simulink model "MPC_control"  (R2018a)
settings: Solver=FixedStepAuto  StartTime=0  StopTime=Tend  FixedStep=0.001  RelTol=5e-3
model workspace (MAT data in the model file):
  A_mu = 10
  B_reff = 8.386
  Cz = 7766.25
  DCT_Param : struct (value not decoded)
  D_reff = 0.25826
  Downshift_Speeds = [9.5625 12.9375 16.3125 19.6875 23.0625 26.4375 29.8125 33.1875 36.5625 39.9375 43.3125 46.6875 ... (28 elements, 4x7)]
  Pedal_Positions = [0.1 0.4 0.5 0.9]
  SUS : struct (value not decoded)
  Upshift_Speeds = [12.9375 16.3125 19.6875 33 26.4375 29.8125 33.1875 52.5 39.9375 43.3125 46.6875 77.25 ... (28 elements, 4x7)]
  VEH : struct (value not decoded)
  V_o = 16.7
  V_xlow = 1
  WH : struct (value not decoded)
  a = 1.4
  alpha_max = 1.5
  alpha_min = -1.5
  b = 1.8
  c_zo = 209651
  epsilon = 0.1
  h = 0.134
  path : struct (value not decoded)
  pio = 220000
  q_Fcx = 0
  q_Fz2 = 15.4
  q_Fzy = 0
  q_reo = 0.9974
  q_sx1 = -0.007764
  q_sx10 = 0.2824
  q_sx11 = 5.349
  q_sx12 = 0
  q_sx13 = 0
  q_sx14 = 0
  q_sx2 = 1.1915
  q_sx3 = 0.013948
  q_sx4 = 4.912
  q_sx5 = 1.02
  q_sx6 = 22.83
  q_sx7 = 0.7104
  q_sx8 = -0.023393
  q_sx9 = 0.6581
  q_sy1 = 0.00702
  q_sy2 = 0
  q_sy3 = 0.001515
  q_sy4 = 8.514e-05
  q_sy5 = 0
  q_sy6 = 0
  q_sy7 = 0.9008
  q_sy8 = -0.4089
  q_v1 = 0.0007742
  q_v2 = 0.04667
  r_Bx1 = 12.531
  r_Bx2 = 9.532
  r_Bx3 = 0
  r_By1 = 10.615
  r_By2 = 7.705
  r_By3 = 3.433e-06
  r_By4 = 0
  r_Cx1 = 1.019
  r_Cy1 = 1.0585
  r_Ex1 = -0.4487
  r_Ex2 = -0.4726
  r_Ey1 = 0.3132
  r_Ey2 = 7.63e-06
  r_Hx1 = 0.0002374
  r_Hy1 = 0.011646
  r_Hy2 = 7.63e-06
  r_Vy1 = 0.05654
  r_Vy2 = 7.63e-06
  r_Vy3 = 0
  r_Vy4 = 99.9
  r_Vy5 = 2
  r_Vy6 = 15.814
  r_o = 0.3135
  vehWidth = 2
  w = 1
symbols that are objects in the model workspace (value not decoded): VEH
undefined symbols (not defined in the file): Cok_1, Cok_2, Cok_3, Cok_4, Cok_5, Cok_6, Cok_7, Cok_8, Cok_9, Cout_1, Cout_2, Cout_3, Cout_4, Cout_5, Cout_6, Cout_7, Cout_8, Cout_9, DiscIntNeverNeededParam, Dout_1, Dout_2, Dout_3, Dout_4, Dout_5, Dout_6, Dout_7, Dout_8, Dout_9, F_1, F_2, F_3, F_4, F_5, F_6, F_7, F_8, F_9, Gd_1, Gd_2, Gd_3, Gd_4, Gd_5, Gd_6, Gd_7, Gd_8, Gd_9, Gok_1, Gok_2, Gok_3, Gok_4, Gok_5, Gok_6, Gok_7, Gok_8, Gok_9, Gsys_2, Gsys_9, Hd_1, Hd_2, Hd_3 ... (+70)
libraries: robotalgslib x10, simulink x5, sim3dlib x2, autolibutils x1, vehdynlibviscommon x1
(part 3 of 5)

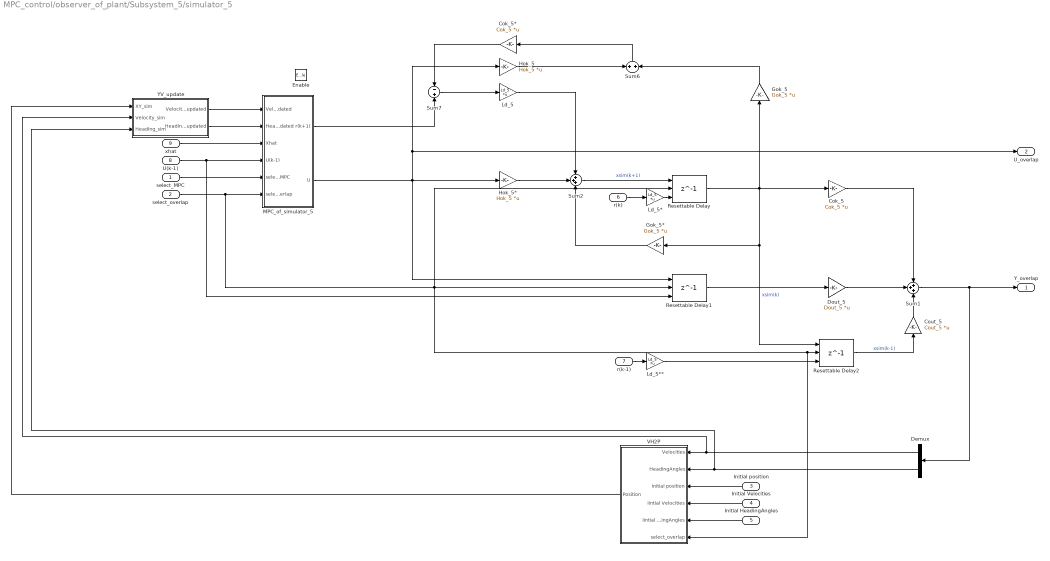
== system MPC_control/observer_of_plant/Subsystem_5/simulator_5 ==
  select_MPC : Inport
  select_overlap : Inport  Port=2
  Initial position : Inport  Port=3
  Initial Velocities : Inport  Port=4
  Initial HeadingAngles : Inport  Port=5
  r(k) : Inport  Port=6
  r(k-1) : Inport  Port=7
  U(k-1) : Inport  Port=8
  xhat : Inport  Port=9
  Enable : EnablePort
  Cok_5 : Gain  Gain=Cok_5  Multiplication=Matrix(K*u) (u vector)
  Cok_5* : Gain  Gain=Cok_5  Multiplication=Matrix(K*u) (u vector)
  Cout_5 : Gain  Gain=Cout_5  Multiplication=Matrix(K*u) (u vector)
  Demux : Demux  Outputs=2
  Dout_5 : Gain  Gain=Dout_5  Multiplication=Matrix(K*u) (u vector)
  Gok_5 : Gain  Gain=Gok_5  Multiplication=Matrix(K*u) (u vector)
  Gok_5* : Gain  Gain=Gok_5  Multiplication=Matrix(K*u) (u vector)
  Hok_5 : Gain  Gain=Hok_5  Multiplication=Matrix(K*u) (u vector)
  Hok_5* : Gain  Gain=Hok_5  Multiplication=Matrix(K*u) (u vector)
  Ld_5 : Gain  Gain=Ld_5  Multiplication=Matrix(K*u) (u vector)
  Ld_5* : Gain  Gain=Ld_5  Multiplication=Matrix(K*u) (u vector)
  Ld_5** : Gain  Gain=Ld_5  Multiplication=Matrix(K*u) (u vector)
  MPC_of_simulator_5 : Subsystem
  Resettable Delay : Delay  DelayLength=1  InitialConditionSource=Input port  ExternalReset=Rising  SampleTime=Ts
      settings: InputPortMap=u0,r5,p4
  Resettable Delay1 : Delay  DelayLength=1  InitialConditionSource=Input port  ExternalReset=Rising  SampleTime=Ts
      settings: InputPortMap=u0,r5,p4
  Resettable Delay2 : Delay  DelayLength=1  InitialConditionSource=Input port  ExternalReset=Rising  SampleTime=Ts
      settings: InputPortMap=u0,r5,p4
  Sum1 : Sum  Inputs=+++
  Sum2 : Sum  Inputs=+++
  Sum6 : Sum
  Sum7 : Sum  Inputs=-+
  VH2P : Subsystem
  YV_update : Subsystem  TreatAsAtomicUnit=on
  Y_overlap : Outport
  U_overlap : Outport  Port=2
  wires:
  Initial position/1 -> VH2P/3(Initial position)
  Sum2/1 -> Resettable Delay/1  "xsim(k+1)"
  Demux/2 -> VH2P/2(HeadingAngles), YV_update/3(Heading_sim)
  Ld_5/1 -> Sum2/1
  Sum7/1 -> Ld_5/1
  Cout_5/1 -> Sum1/3
  MPC_of_simulator_5/2(U) -> Hok_5*/1, Resettable Delay1/1, Hok_5/1, U_overlap/1
  Hok_5*/1 -> Sum2/2
  Gok_5*/1 -> Sum2/3
  Resettable Delay2/1 -> Cout_5/1  "xsim(k-1)"
  VH2P/1(Position) -> YV_update/1(XY_sim)
  Demux/1 -> YV_update/2(Velocity_sim), VH2P/1(Velocities)
  Resettable Delay/1 -> Gok_5*/1, Resettable Delay2/1, Gok_5/1, Cok_5/1  "xsim(k)"
  Hok_5/1 -> Sum6/1
  Sum6/1 -> Cok_5*/1
  Dout_5/1 -> Sum1/2
  Resettable Delay1/1 -> Dout_5/1
  Cok_5/1 -> Sum1/1
  YV_update/2(Heading_updated) -> MPC_of_simulator_5/2(Heading_updated)
  YV_update/1(Velocity_updated) -> MPC_of_simulator_5/1(Velocity_updated)
  r(k)/1 -> Ld_5*/1
  Ld_5*/1 -> Resettable Delay/3
  U(k-1)/1 -> MPC_of_simulator_5/4(U(k-1)), Resettable Delay1/3
  r(k-1)/1 -> Ld_5**/1
  Ld_5**/1 -> Resettable Delay2/3
  Initial Velocities/1 -> VH2P/4(Iintial Velocities)
  Initial HeadingAngles/1 -> VH2P/5(Iintial HeadingAngles)
  select_overlap/1 -> MPC_of_simulator_5/6(select_overlap), Resettable Delay/2, VH2P/6(select_overlap), Resettable Delay2/2, Resettable Delay1/2
  Gok_5/1 -> Sum6/2
  Cok_5*/1 -> Sum7/1
  select_MPC/1 -> MPC_of_simulator_5/5(select_MPC)
  Sum1/1 -> Y_overlap/1, Demux/1
  MPC_of_simulator_5/1(r(k+1)) -> Sum7/2
  xhat/1 -> MPC_of_simulator_5/3(Xhat)

== system MPC_control/observer_of_plant/Subsystem_6/observer_of_simulator_6 ==
  select_overlap : Inport
  U_overlap : Inport  Port=2
  U : Inport  Port=3
  U(k-1) : Inport  Port=4
  Y_overlap : Inport  Port=5
  Y : Inport  Port=6
  r(k-1) : Inport  Port=7
  Cok_6 : Gain  Gain=Cok_6  Multiplication=Matrix(K*u) (u vector)
  Cok_6* : Gain  Gain=Cok_6  Multiplication=Matrix(K*u) (u vector)
  Delay : Delay  DelayLength=1  InitialConditionSource=Input port  InitialCondition=0  ExternalReset=Rising  SampleTime=Ts
      settings: InputPortMap=u0,r5,p4
  Delay1 : Delay  DelayLength=1  InitialConditionSource=Input port  InitialCondition=0  ExternalReset=Rising  SampleTime=Ts
      settings: InputPortMap=u0,r5,p4
  Gd_6 : Gain  Gain=Gd_6  Multiplication=Matrix(K*u) (u vector)
  Gok_6 : Gain  Gain=Gok_6  Multiplication=Matrix(K*u) (u vector)
  Hd_6 : Gain  Gain=Hd_6  Multiplication=Matrix(K*u) (u vector)
  Hok_6 : Gain  Gain=Hok_6  Multiplication=Matrix(K*u) (u vector)
  Ld_6 : Gain  Gain=Ld_6  Multiplication=Matrix(K*u) (u vector)
  Ld_6* : Gain  Gain=Ld_6  Multiplication=Matrix(K*u) (u vector)
  Sum : Sum  Inputs=|-+
  Sum1 : Sum
  Sum2 : Sum  Inputs=|-+
  Sum4 : Sum  Inputs=+++
  Switch1 : Switch  Threshold=1
  Switch2 : Switch  Threshold=1
  xhat : Outport
  sye : Outport  Port=2
  ope : Outport  Port=3
  wires:
  Hd_6/1 -> Sum4/2
  Ld_6/1 -> Sum4/1
  Delay1/1 -> Hok_6/1, Hd_6/1
  U_overlap/1 -> Switch2/1
  Gd_6/1 -> Sum4/3
  U/1 -> Switch2/3
  Delay/1 -> Gok_6/1, Gd_6/1
  Y_overlap/1 -> Switch1/1
  U(k-1)/1 -> Delay1/3
  select_overlap/1 -> Delay/2, Delay1/2, Switch2/2, Switch1/2
  r(k-1)/1 -> Ld_6*/1
  Switch1/1 -> Ld_6/1
  Switch2/1 -> Delay1/1
  Ld_6*/1 -> Delay/3
  Sum2/1 -> sye/1
  Gok_6/1 -> Sum1/1
  Cok_6/1 -> Sum/1
  Hok_6/1 -> Sum1/2
  Y/1 -> Sum/2, Sum2/2, Switch1/3
  Cok_6*/1 -> Sum2/1
  Sum1/1 -> Cok_6*/1
  Sum/1 -> ope/1
  Sum4/1 -> xhat/1, Cok_6/1, Delay/1  "xhat"

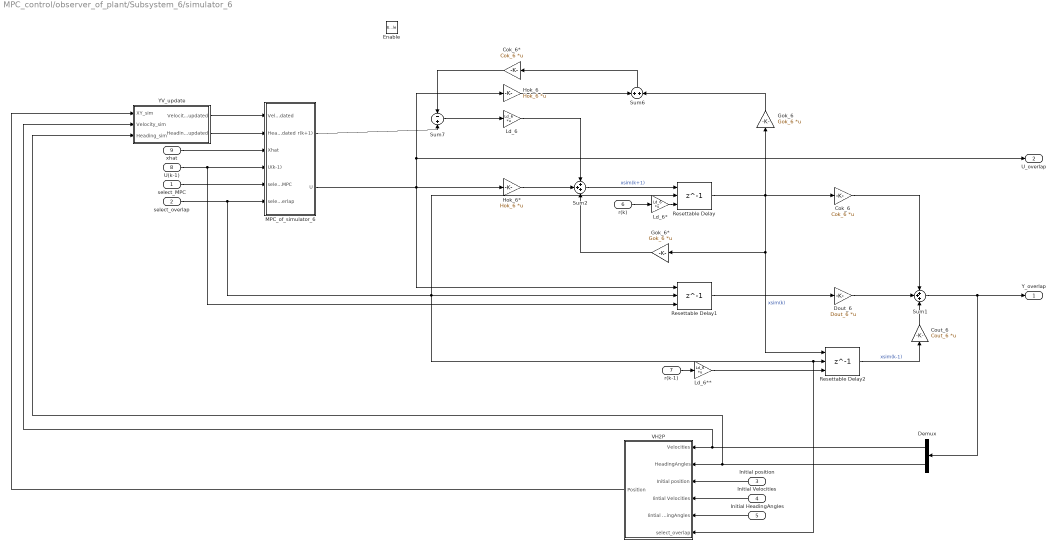
== system MPC_control/observer_of_plant/Subsystem_6/simulator_6 ==
  select_MPC : Inport
  select_overlap : Inport  Port=2
  Initial position : Inport  Port=3
  Initial Velocities : Inport  Port=4
  Initial HeadingAngles : Inport  Port=5
  r(k) : Inport  Port=6
  r(k-1) : Inport  Port=7
  U(k-1) : Inport  Port=8
  xhat : Inport  Port=9
  Enable : EnablePort
  Cok_6 : Gain  Gain=Cok_6  Multiplication=Matrix(K*u) (u vector)
  Cok_6* : Gain  Gain=Cok_6  Multiplication=Matrix(K*u) (u vector)
  Cout_6 : Gain  Gain=Cout_6  Multiplication=Matrix(K*u) (u vector)
  Demux : Demux  Outputs=2
  Dout_6 : Gain  Gain=Dout_6  Multiplication=Matrix(K*u) (u vector)
  Gok_6 : Gain  Gain=Gok_6  Multiplication=Matrix(K*u) (u vector)
  Gok_6* : Gain  Gain=Gok_6  Multiplication=Matrix(K*u) (u vector)
  Hok_6 : Gain  Gain=Hok_6  Multiplication=Matrix(K*u) (u vector)
  Hok_6* : Gain  Gain=Hok_6  Multiplication=Matrix(K*u) (u vector)
  Ld_6 : Gain  Gain=Ld_6  Multiplication=Matrix(K*u) (u vector)
  Ld_6* : Gain  Gain=Ld_6  Multiplication=Matrix(K*u) (u vector)
  Ld_6** : Gain  Gain=Ld_6  Multiplication=Matrix(K*u) (u vector)
  MPC_of_simulator_6 : Subsystem
  Resettable Delay : Delay  DelayLength=1  InitialConditionSource=Input port  ExternalReset=Rising  SampleTime=Ts
      settings: InputPortMap=u0,r5,p4
  Resettable Delay1 : Delay  DelayLength=1  InitialConditionSource=Input port  ExternalReset=Rising  SampleTime=Ts
      settings: InputPortMap=u0,r5,p4
  Resettable Delay2 : Delay  DelayLength=1  InitialConditionSource=Input port  ExternalReset=Rising  SampleTime=Ts
      settings: InputPortMap=u0,r5,p4
  Sum1 : Sum  Inputs=+++
  Sum2 : Sum  Inputs=+++
  Sum6 : Sum
  Sum7 : Sum  Inputs=-+
  VH2P : Subsystem
  YV_update : Subsystem  TreatAsAtomicUnit=on
  Y_overlap : Outport
  U_overlap : Outport  Port=2
  wires:
  Initial position/1 -> VH2P/3(Initial position)
  Sum2/1 -> Resettable Delay/1  "xsim(k+1)"
  Demux/2 -> VH2P/2(HeadingAngles), YV_update/3(Heading_sim)
  Ld_6/1 -> Sum2/1
  Sum7/1 -> Ld_6/1
  Cout_6/1 -> Sum1/3
  MPC_of_simulator_6/2(U) -> Hok_6*/1, Hok_6/1, U_overlap/1, Resettable Delay1/1
  Hok_6*/1 -> Sum2/2
  Gok_6*/1 -> Sum2/3
  Resettable Delay2/1 -> Cout_6/1  "xsim(k-1)"
  VH2P/1(Position) -> YV_update/1(XY_sim)
  Demux/1 -> YV_update/2(Velocity_sim), VH2P/1(Velocities)
  Resettable Delay/1 -> Gok_6*/1, Resettable Delay2/1, Gok_6/1, Cok_6/1  "xsim(k)"
  Hok_6/1 -> Sum6/1
  Sum6/1 -> Cok_6*/1
  Dout_6/1 -> Sum1/2
  Resettable Delay1/1 -> Dout_6/1
  Cok_6/1 -> Sum1/1
  YV_update/2(Heading_updated) -> MPC_of_simulator_6/2(Heading_updated)
  YV_update/1(Velocity_updated) -> MPC_of_simulator_6/1(Velocity_updated)
  r(k)/1 -> Ld_6*/1
  Ld_6*/1 -> Resettable Delay/3
  U(k-1)/1 -> MPC_of_simulator_6/4(U(k-1)), Resettable Delay1/3
  r(k-1)/1 -> Ld_6**/1
  Ld_6**/1 -> Resettable Delay2/3
  Initial Velocities/1 -> VH2P/4(Iintial Velocities)
  Initial HeadingAngles/1 -> VH2P/5(Iintial HeadingAngles)
  select_overlap/1 -> MPC_of_simulator_6/6(select_overlap), Resettable Delay/2, VH2P/6(select_overlap), Resettable Delay2/2, Resettable Delay1/2
  Gok_6/1 -> Sum6/2
  Cok_6*/1 -> Sum7/1
  select_MPC/1 -> MPC_of_simulator_6/5(select_MPC)
  Sum1/1 -> Y_overlap/1, Demux/1
  MPC_of_simulator_6/1(r(k+1)) -> Sum7/2
  xhat/1 -> MPC_of_simulator_6/3(Xhat)

== system MPC_control/observer_of_plant/Subsystem_7/observer_of_simulator_7 ==
  select_overlap : Inport
  U_overlap : Inport  Port=2
  U : Inport  Port=3
  U(k-1) : Inport  Port=4
  Y_overlap : Inport  Port=5
  Y : Inport  Port=6
  r(k-1) : Inport  Port=7
  Cok_7 : Gain  Gain=Cok_7  Multiplication=Matrix(K*u) (u vector)
  Cok_7* : Gain  Gain=Cok_7  Multiplication=Matrix(K*u) (u vector)
  Delay : Delay  DelayLength=1  InitialConditionSource=Input port  InitialCondition=0  ExternalReset=Rising  SampleTime=Ts
      settings: InputPortMap=u0,r5,p4
  Delay1 : Delay  DelayLength=1  InitialConditionSource=Input port  InitialCondition=0  ExternalReset=Rising  SampleTime=Ts
      settings: InputPortMap=u0,r5,p4
  Gd_7 : Gain  Gain=Gd_7  Multiplication=Matrix(K*u) (u vector)
  Gok_7 : Gain  Gain=Gok_7  Multiplication=Matrix(K*u) (u vector)
  Hd_7 : Gain  Gain=Hd_7  Multiplication=Matrix(K*u) (u vector)
  Hok_7 : Gain  Gain=Hok_7  Multiplication=Matrix(K*u) (u vector)
  Ld_7 : Gain  Gain=Ld_7  Multiplication=Matrix(K*u) (u vector)
  Ld_7* : Gain  Gain=Ld_7  Multiplication=Matrix(K*u) (u vector)
  Sum : Sum  Inputs=|-+
  Sum1 : Sum
  Sum2 : Sum  Inputs=|-+
  Sum4 : Sum  Inputs=+++
  Switch1 : Switch  Threshold=1
  Switch2 : Switch  Threshold=1
  xhat : Outport
  sye : Outport  Port=2
  ope : Outport  Port=3
  wires:
  Hd_7/1 -> Sum4/2
  Ld_7/1 -> Sum4/1
  U_overlap/1 -> Switch2/1
  Gd_7/1 -> Sum4/3
  U/1 -> Switch2/3
  Y_overlap/1 -> Switch1/1
  U(k-1)/1 -> Delay1/3
  select_overlap/1 -> Delay/2, Delay1/2, Switch2/2, Switch1/2
  r(k-1)/1 -> Ld_7*/1
  Switch1/1 -> Ld_7/1
  Switch2/1 -> Delay1/1
  Ld_7*/1 -> Delay/3
  Delay/1 -> Gok_7/1, Gd_7/1
  Sum2/1 -> sye/1
  Sum/1 -> ope/1
  Cok_7/1 -> Sum/1
  Hok_7/1 -> Sum1/2
  Delay1/1 -> Hok_7/1, Hd_7/1
  Gok_7/1 -> Sum1/1
  Y/1 -> Sum/2, Sum2/2, Switch1/3
  Cok_7*/1 -> Sum2/1
  Sum1/1 -> Cok_7*/1
  Sum4/1 -> xhat/1, Cok_7/1, Delay/1  "xhat"

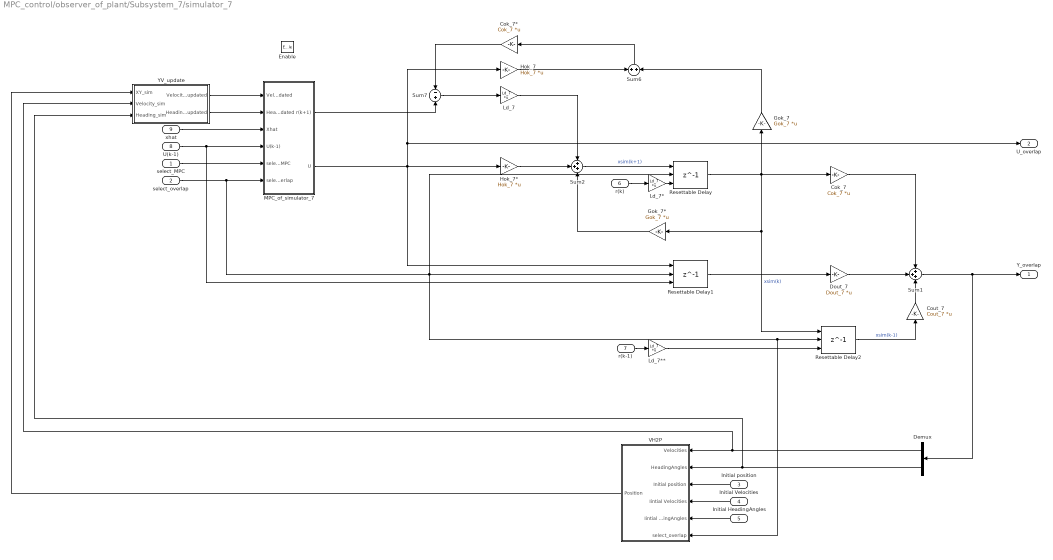
== system MPC_control/observer_of_plant/Subsystem_7/simulator_7 ==
  select_MPC : Inport
  select_overlap : Inport  Port=2
  Initial position : Inport  Port=3
  Initial Velocities : Inport  Port=4
  Initial HeadingAngles : Inport  Port=5
  r(k) : Inport  Port=6
  r(k-1) : Inport  Port=7
  U(k-1) : Inport  Port=8
  xhat : Inport  Port=9
  Enable : EnablePort
  Cok_7 : Gain  Gain=Cok_7  Multiplication=Matrix(K*u) (u vector)
  Cok_7* : Gain  Gain=Cok_7  Multiplication=Matrix(K*u) (u vector)
  Cout_7 : Gain  Gain=Cout_7  Multiplication=Matrix(K*u) (u vector)
  Demux : Demux  Outputs=2
  Dout_7 : Gain  Gain=Dout_7  Multiplication=Matrix(K*u) (u vector)
  Gok_7 : Gain  Gain=Gok_7  Multiplication=Matrix(K*u) (u vector)
  Gok_7* : Gain  Gain=Gok_7  Multiplication=Matrix(K*u) (u vector)
  Hok_7 : Gain  Gain=Hok_7  Multiplication=Matrix(K*u) (u vector)
  Hok_7* : Gain  Gain=Hok_7  Multiplication=Matrix(K*u) (u vector)
  Ld_7 : Gain  Gain=Ld_7  Multiplication=Matrix(K*u) (u vector)
  Ld_7* : Gain  Gain=Ld_7  Multiplication=Matrix(K*u) (u vector)
  Ld_7** : Gain  Gain=Ld_7  Multiplication=Matrix(K*u) (u vector)
  MPC_of_simulator_7 : Subsystem
  Resettable Delay : Delay  DelayLength=1  InitialConditionSource=Input port  ExternalReset=Rising  SampleTime=Ts
      settings: InputPortMap=u0,r5,p4
  Resettable Delay1 : Delay  DelayLength=1  InitialConditionSource=Input port  ExternalReset=Rising  SampleTime=Ts
      settings: InputPortMap=u0,r5,p4
  Resettable Delay2 : Delay  DelayLength=1  InitialConditionSource=Input port  ExternalReset=Rising  SampleTime=Ts
      settings: InputPortMap=u0,r5,p4
  Sum1 : Sum  Inputs=+++
  Sum2 : Sum  Inputs=+++
  Sum6 : Sum
  Sum7 : Sum  Inputs=-+
  VH2P : Subsystem
  YV_update : Subsystem  TreatAsAtomicUnit=on
  Y_overlap : Outport
  U_overlap : Outport  Port=2
  wires:
  Sum2/1 -> Resettable Delay/1  "xsim(k+1)"
  Demux/2 -> VH2P/2(HeadingAngles), YV_update/3(Heading_sim)
  Ld_7/1 -> Sum2/1
  Sum7/1 -> Ld_7/1
  Cout_7/1 -> Sum1/3
  MPC_of_simulator_7/2(U) -> Hok_7/1, U_overlap/1, Hok_7*/1, Resettable Delay1/1
  Hok_7*/1 -> Sum2/2
  Gok_7*/1 -> Sum2/3
  Resettable Delay2/1 -> Cout_7/1  "xsim(k-1)"
  VH2P/1(Position) -> YV_update/1(XY_sim)
  Demux/1 -> YV_update/2(Velocity_sim), VH2P/1(Velocities)
  Resettable Delay/1 -> Gok_7*/1, Resettable Delay2/1, Gok_7/1, Cok_7/1  "xsim(k)"
  Hok_7/1 -> Sum6/1
  Sum6/1 -> Cok_7*/1
  Dout_7/1 -> Sum1/2
  Resettable Delay1/1 -> Dout_7/1
  Cok_7/1 -> Sum1/1
  YV_update/2(Heading_updated) -> MPC_of_simulator_7/2(Heading_updated)
  YV_update/1(Velocity_updated) -> MPC_of_simulator_7/1(Velocity_updated)
  r(k)/1 -> Ld_7*/1
  Ld_7*/1 -> Resettable Delay/3
  U(k-1)/1 -> MPC_of_simulator_7/4(U(k-1)), Resettable Delay1/3
  r(k-1)/1 -> Ld_7**/1
  Ld_7**/1 -> Resettable Delay2/3
  select_overlap/1 -> MPC_of_simulator_7/6(select_overlap), Resettable Delay/2, Resettable Delay2/2, VH2P/6(select_overlap), Resettable Delay1/2
  Gok_7/1 -> Sum6/2
  Cok_7*/1 -> Sum7/1
  select_MPC/1 -> MPC_of_simulator_7/5(select_MPC)
  Sum1/1 -> Demux/1, Y_overlap/1
  MPC_of_simulator_7/1(r(k+1)) -> Sum7/2
  Initial position/1 -> VH2P/3(Initial position)
  Initial Velocities/1 -> VH2P/4(Iintial Velocities)
  Initial HeadingAngles/1 -> VH2P/5(Iintial HeadingAngles)
  xhat/1 -> MPC_of_simulator_7/3(Xhat)

== system MPC_control/observer_of_plant/Subsystem_8/observer_of_simulator_8 ==
  select_overlap : Inport
  U_overlap : Inport  Port=2
  U : Inport  Port=3
  U(k-1) : Inport  Port=4
  Y_overlap : Inport  Port=5
  Y : Inport  Port=6
  r(k-1) : Inport  Port=7
  Cok_8 : Gain  Gain=Cok_8  Multiplication=Matrix(K*u) (u vector)
  Cok_8* : Gain  Gain=Cok_8  Multiplication=Matrix(K*u) (u vector)
  Delay : Delay  DelayLength=1  InitialConditionSource=Input port  InitialCondition=0  ExternalReset=Rising  SampleTime=Ts
      settings: InputPortMap=u0,r5,p4
  Delay1 : Delay  DelayLength=1  InitialConditionSource=Input port  InitialCondition=0  ExternalReset=Rising  SampleTime=Ts
      settings: InputPortMap=u0,r5,p4
  Gd_8 : Gain  Gain=Gd_8  Multiplication=Matrix(K*u) (u vector)
  Gok_8 : Gain  Gain=Gok_8  Multiplication=Matrix(K*u) (u vector)
  Hd_8 : Gain  Gain=Hd_8  Multiplication=Matrix(K*u) (u vector)
  Hok_8 : Gain  Gain=Hok_8  Multiplication=Matrix(K*u) (u vector)
  Ld_8 : Gain  Gain=Ld_8  Multiplication=Matrix(K*u) (u vector)
  Ld_8* : Gain  Gain=Ld_8  Multiplication=Matrix(K*u) (u vector)
  Sum : Sum  Inputs=|-+
  Sum1 : Sum
  Sum2 : Sum  Inputs=|-+
  Sum4 : Sum  Inputs=+++
  Switch1 : Switch  Threshold=1
  Switch2 : Switch  Threshold=1
  xhat : Outport
  sye : Outport  Port=2
  ope : Outport  Port=3
  wires:
  Hd_8/1 -> Sum4/2
  Ld_8/1 -> Sum4/1
  U_overlap/1 -> Switch2/1
  Gd_8/1 -> Sum4/3
  U/1 -> Switch2/3
  Y_overlap/1 -> Switch1/1
  U(k-1)/1 -> Delay1/3
  select_overlap/1 -> Delay/2, Delay1/2, Switch2/2, Switch1/2
  r(k-1)/1 -> Ld_8*/1
  Switch1/1 -> Ld_8/1
  Switch2/1 -> Delay1/1
  Ld_8*/1 -> Delay/3
  Delay/1 -> Gok_8/1, Gd_8/1
  Sum2/1 -> sye/1
  Sum/1 -> ope/1
  Cok_8/1 -> Sum/1
  Hok_8/1 -> Sum1/2
  Delay1/1 -> Hok_8/1, Hd_8/1
  Gok_8/1 -> Sum1/1
  Y/1 -> Sum/2, Sum2/2, Switch1/3
  Cok_8*/1 -> Sum2/1
  Sum1/1 -> Cok_8*/1
  Sum4/1 -> xhat/1, Cok_8/1, Delay/1  "xhat"

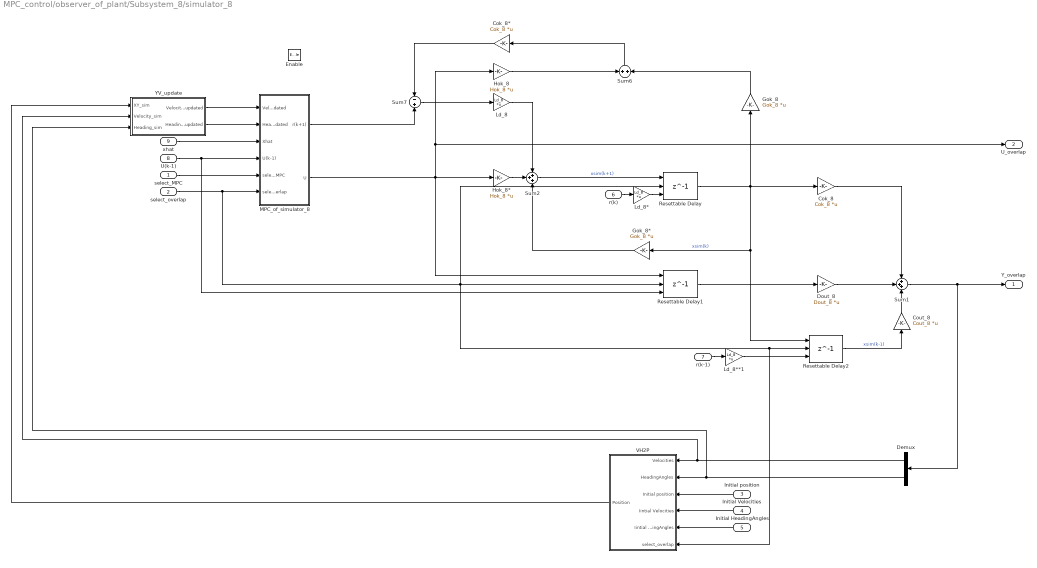
== system MPC_control/observer_of_plant/Subsystem_8/simulator_8 ==
  select_MPC : Inport
  select_overlap : Inport  Port=2
  Initial position : Inport  Port=3
  Initial Velocities : Inport  Port=4
  Initial HeadingAngles : Inport  Port=5
  r(k) : Inport  Port=6
  r(k-1) : Inport  Port=7
  U(k-1) : Inport  Port=8
  xhat : Inport  Port=9
  Enable : EnablePort
  Cok_8 : Gain  Gain=Cok_8  Multiplication=Matrix(K*u) (u vector)
  Cok_8* : Gain  Gain=Cok_8  Multiplication=Matrix(K*u) (u vector)
  Cout_8 : Gain  Gain=Cout_8  Multiplication=Matrix(K*u) (u vector)
  Demux : Demux  Outputs=2
  Dout_8 : Gain  Gain=Dout_8  Multiplication=Matrix(K*u) (u vector)
  Gok_8 : Gain  Gain=Gok_8  Multiplication=Matrix(K*u) (u vector)
  Gok_8* : Gain  Gain=Gok_8  Multiplication=Matrix(K*u) (u vector)
  Hok_8 : Gain  Gain=Hok_8  Multiplication=Matrix(K*u) (u vector)
  Hok_8* : Gain  Gain=Hok_8  Multiplication=Matrix(K*u) (u vector)
  Ld_8 : Gain  Gain=Ld_8  Multiplication=Matrix(K*u) (u vector)
  Ld_8* : Gain  Gain=Ld_8  Multiplication=Matrix(K*u) (u vector)
  Ld_8**1 : Gain  Gain=Ld_8  Multiplication=Matrix(K*u) (u vector)
  MPC_of_simulator_8 : Subsystem
  Resettable Delay : Delay  DelayLength=1  InitialConditionSource=Input port  ExternalReset=Rising  SampleTime=Ts
      settings: InputPortMap=u0,r5,p4
  Resettable Delay1 : Delay  DelayLength=1  InitialConditionSource=Input port  ExternalReset=Rising  SampleTime=Ts
      settings: InputPortMap=u0,r5,p4
  Resettable Delay2 : Delay  DelayLength=1  InitialConditionSource=Input port  ExternalReset=Rising  SampleTime=Ts
      settings: InputPortMap=u0,r5,p4
  Sum1 : Sum  Inputs=+++
  Sum2 : Sum  Inputs=+++
  Sum6 : Sum
  Sum7 : Sum  Inputs=-+
  VH2P : Subsystem
  YV_update : Subsystem  TreatAsAtomicUnit=on
  Y_overlap : Outport
  U_overlap : Outport  Port=2
  wires:
  Sum2/1 -> Resettable Delay/1  "xsim(k+1)"
  Demux/2 -> VH2P/2(HeadingAngles), YV_update/3(Heading_sim)
  Ld_8/1 -> Sum2/1
  Sum7/1 -> Ld_8/1
  Cout_8/1 -> Sum1/3
  MPC_of_simulator_8/2(U) -> Hok_8/1, U_overlap/1, Hok_8*/1, Resettable Delay1/1
  Hok_8*/1 -> Sum2/2
  Gok_8*/1 -> Sum2/3
  VH2P/1(Position) -> YV_update/1(XY_sim)
  Demux/1 -> VH2P/1(Velocities), YV_update/2(Velocity_sim)
  Resettable Delay/1 -> Resettable Delay2/1, Gok_8*/1, Gok_8/1, Cok_8/1  "xsim(k)"
  Hok_8/1 -> Sum6/1
  Sum6/1 -> Cok_8*/1
  Dout_8/1 -> Sum1/2
  Resettable Delay1/1 -> Dout_8/1
  Cok_8/1 -> Sum1/1
  YV_update/2(Heading_updated) -> MPC_of_simulator_8/2(Heading_updated)
  YV_update/1(Velocity_updated) -> MPC_of_simulator_8/1(Velocity_updated)
  select_overlap/1 -> MPC_of_simulator_8/6(select_overlap), Resettable Delay2/2, VH2P/6(select_overlap), Resettable Delay/2, Resettable Delay1/2
  Gok_8/1 -> Sum6/2
  Cok_8*/1 -> Sum7/1
  select_MPC/1 -> MPC_of_simulator_8/5(select_MPC)
  Sum1/1 -> Demux/1, Y_overlap/1
  MPC_of_simulator_8/1(r(k+1)) -> Sum7/2
  Resettable Delay2/1 -> Cout_8/1  "xsim(k-1)"
  Ld_8**1/1 -> Resettable Delay2/3
  U(k-1)/1 -> Resettable Delay1/3, MPC_of_simulator_8/4(U(k-1))
  r(k)/1 -> Ld_8*/1
  Ld_8*/1 -> Resettable Delay/3
  r(k-1)/1 -> Ld_8**1/1
  Initial Velocities/1 -> VH2P/4(Iintial Velocities)
  Initial position/1 -> VH2P/3(Initial position)
  Initial HeadingAngles/1 -> VH2P/5(Iintial HeadingAngles)
  xhat/1 -> MPC_of_simulator_8/3(Xhat)

== system MPC_control/observer_of_plant/Subsystem_9/observer_of_simulator_9 ==
  select_overlap : Inport
  U_overlap : Inport  Port=2
  U : Inport  Port=3
  U(k-1) : Inport  Port=4
  Y_overlap : Inport  Port=5
  Y : Inport  Port=6
  r(k-1) : Inport  Port=7
  Cok_9 : Gain  Gain=Cok_9  Multiplication=Matrix(K*u) (u vector)
  Cok_9* : Gain  Gain=Cok_9  Multiplication=Matrix(K*u) (u vector)
  Delay : Delay  DelayLength=1  InitialConditionSource=Input port  InitialCondition=0  ExternalReset=Rising  SampleTime=Ts
      settings: InputPortMap=u0,r5,p4
  Delay1 : Delay  DelayLength=1  InitialConditionSource=Input port  InitialCondition=0  ExternalReset=Rising  SampleTime=Ts
      settings: InputPortMap=u0,r5,p4
  Gd_9 : Gain  Gain=Gd_9  Multiplication=Matrix(K*u) (u vector)
  Gok_9 : Gain  Gain=Gok_9  Multiplication=Matrix(K*u) (u vector)
  Hd_9 : Gain  Gain=Hd_9  Multiplication=Matrix(K*u) (u vector)
  Hok_9 : Gain  Gain=Hok_9  Multiplication=Matrix(K*u) (u vector)
  Ld_9 : Gain  Gain=Ld_9  Multiplication=Matrix(K*u) (u vector)
  Ld_9* : Gain  Gain=Ld_9  Multiplication=Matrix(K*u) (u vector)
  Sum : Sum  Inputs=|-+
  Sum1 : Sum
  Sum2 : Sum  Inputs=|-+
  Sum4 : Sum  Inputs=+++
  Switch1 : Switch  Threshold=1
  Switch2 : Switch  Threshold=1
  xhat : Outport
  sye : Outport  Port=2
  ope : Outport  Port=3
  wires:
  Hd_9/1 -> Sum4/2
  Ld_9/1 -> Sum4/1
  U_overlap/1 -> Switch2/1
  Gd_9/1 -> Sum4/3
  U/1 -> Switch2/3
  Y_overlap/1 -> Switch1/1
  U(k-1)/1 -> Delay1/3
  select_overlap/1 -> Delay/2, Delay1/2, Switch2/2, Switch1/2
  r(k-1)/1 -> Ld_9*/1
  Switch1/1 -> Ld_9/1
  Switch2/1 -> Delay1/1
  Ld_9*/1 -> Delay/3
  Delay/1 -> Gok_9/1, Gd_9/1
  Sum2/1 -> sye/1
  Sum/1 -> ope/1
  Cok_9/1 -> Sum/1
  Hok_9/1 -> Sum1/2
  Delay1/1 -> Hok_9/1, Hd_9/1
  Gok_9/1 -> Sum1/1
  Y/1 -> Sum/2, Sum2/2, Switch1/3
  Cok_9*/1 -> Sum2/1
  Sum1/1 -> Cok_9*/1
  Sum4/1 -> xhat/1, Cok_9/1, Delay/1  "xhat"

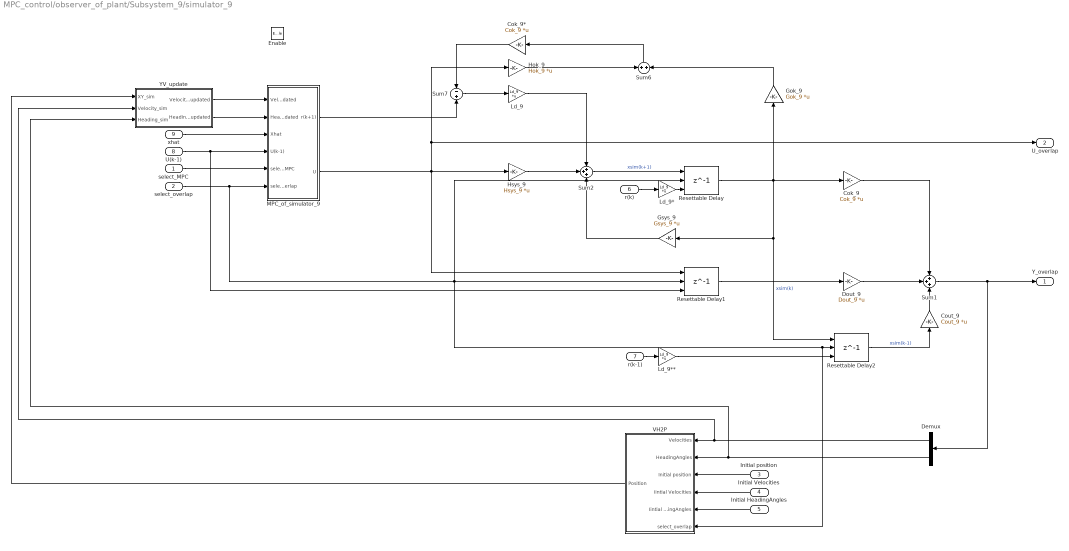
== system MPC_control/observer_of_plant/Subsystem_9/simulator_9 ==
  select_MPC : Inport
  select_overlap : Inport  Port=2
  Initial position : Inport  Port=3
  Initial Velocities : Inport  Port=4
  Initial HeadingAngles : Inport  Port=5
  r(k) : Inport  Port=6
  r(k-1) : Inport  Port=7
  U(k-1) : Inport  Port=8
  xhat : Inport  Port=9
  Enable : EnablePort
  Cok_9 : Gain  Gain=Cok_9  Multiplication=Matrix(K*u) (u vector)
  Cok_9* : Gain  Gain=Cok_9  Multiplication=Matrix(K*u) (u vector)
  Cout_9 : Gain  Gain=Cout_9  Multiplication=Matrix(K*u) (u vector)
  Demux : Demux  Outputs=2
  Dout_9 : Gain  Gain=Dout_9  Multiplication=Matrix(K*u) (u vector)
  Gok_9 : Gain  Gain=Gok_9  Multiplication=Matrix(K*u) (u vector)
  Gsys_9 : Gain  Gain=Gsys_9  Multiplication=Matrix(K*u) (u vector)
  Hok_9 : Gain  Gain=Hok_9  Multiplication=Matrix(K*u) (u vector)
  Hsys_9 : Gain  Gain=Hsys_9  Multiplication=Matrix(K*u) (u vector)
  Ld_9 : Gain  Gain=Ld_9  Multiplication=Matrix(K*u) (u vector)
  Ld_9* : Gain  Gain=Ld_9  Multiplication=Matrix(K*u) (u vector)
  Ld_9** : Gain  Gain=Ld_9  Multiplication=Matrix(K*u) (u vector)
  MPC_of_simulator_9 : Subsystem
  Resettable Delay : Delay  DelayLength=1  InitialConditionSource=Input port  ExternalReset=Rising  SampleTime=Ts
      settings: InputPortMap=u0,r5,p4
  Resettable Delay1 : Delay  DelayLength=1  InitialConditionSource=Input port  ExternalReset=Rising  SampleTime=Ts
      settings: InputPortMap=u0,r5,p4
  Resettable Delay2 : Delay  DelayLength=1  InitialConditionSource=Input port  ExternalReset=Rising  SampleTime=Ts
      settings: InputPortMap=u0,r5,p4
  Sum1 : Sum  Inputs=+++
  Sum2 : Sum  Inputs=+++
  Sum6 : Sum
  Sum7 : Sum  Inputs=-+
  VH2P : Subsystem
  YV_update : Subsystem  TreatAsAtomicUnit=on
  Y_overlap : Outport
  U_overlap : Outport  Port=2
  wires:
  Initial position/1 -> VH2P/3(Initial position)
  Sum2/1 -> Resettable Delay/1  "xsim(k+1)"
  Demux/2 -> VH2P/2(HeadingAngles), YV_update/3(Heading_sim)
  Ld_9/1 -> Sum2/1
  Sum7/1 -> Ld_9/1
  Cout_9/1 -> Sum1/3
  MPC_of_simulator_9/2(U) -> Hok_9/1, U_overlap/1, Resettable Delay1/1, Hsys_9/1
  Hsys_9/1 -> Sum2/2
  Gsys_9/1 -> Sum2/3
  Resettable Delay2/1 -> Cout_9/1  "xsim(k-1)"
  VH2P/1(Position) -> YV_update/1(XY_sim)
  Demux/1 -> YV_update/2(Velocity_sim), VH2P/1(Velocities)
  Resettable Delay/1 -> Gsys_9/1, Resettable Delay2/1, Gok_9/1, Cok_9/1  "xsim(k)"
  Hok_9/1 -> Sum6/1
  Sum6/1 -> Cok_9*/1
  Dout_9/1 -> Sum1/2
  Resettable Delay1/1 -> Dout_9/1
  Cok_9/1 -> Sum1/1
  YV_update/2(Heading_updated) -> MPC_of_simulator_9/2(Heading_updated)
  xhat/1 -> MPC_of_simulator_9/3(Xhat)
  YV_update/1(Velocity_updated) -> MPC_of_simulator_9/1(Velocity_updated)
  r(k)/1 -> Ld_9*/1
  Ld_9*/1 -> Resettable Delay/3
  U(k-1)/1 -> MPC_of_simulator_9/4(U(k-1)), Resettable Delay1/3
  r(k-1)/1 -> Ld_9**/1
  Ld_9**/1 -> Resettable Delay2/3
  Initial Velocities/1 -> VH2P/4(Iintial Velocities)
  Initial HeadingAngles/1 -> VH2P/5(Iintial HeadingAngles)
  select_overlap/1 -> MPC_of_simulator_9/6(select_overlap), Resettable Delay/2, VH2P/6(select_overlap), Resettable Delay2/2, Resettable Delay1/2
  Gok_9/1 -> Sum6/2
  Cok_9*/1 -> Sum7/1
  select_MPC/1 -> MPC_of_simulator_9/5(select_MPC)
  Sum1/1 -> Demux/1, Y_overlap/1
  MPC_of_simulator_9/1(r(k+1)) -> Sum7/2

== system MPC_control/Controllers/Brake Controller/Brake Pressure Control/Bang Bang ABS ==
  Pref : Inport
  xdot : Inport  Port=2
  <Kappa> : Inport  Port=3
  Abs : Abs
  Add : Sum  Inputs=-+
  Bang-bang controller : Subsystem  mask(Sign){}
      mask help: y = sign(x)
      mask Help: Sign Function:\n\t\t\ty = 1 if x > 0\n\t\t\ty = 0 if x = 0\n\t\t\ty = -1 if x < 0
      mask Display: plot(-50,-50,50,50,[-50,50],[0,0],[0,0],[-50,50],[-40,0],[-30,-30],[0,40],[30,30])
  Compare To Constant : simulink/Logic and Bit Operations/Compare To Constant  relop=>=  const=.2  OutDataTypeStr=boolean
  Compare To Constant1 : simulink/Logic and Bit Operations/Compare To Constant  relop=>=  const=.75  OutDataTypeStr=boolean
  Compare To Constant2 : simulink/Logic and Bit Operations/Compare To Constant  relop=>=  const=.5  OutDataTypeStr=boolean
  Constant : Constant  Value=.25
  Debounce : autolibutils/Debounce  DbcOn_Cnts=.1*.001  DbcOff_Cnts=.1*.001  aMode=aMode
      settings: SourceProductName=Powertrain Blockset  SourceProductBaseCode=PW
  Gain : Gain  Gain=200
  Logical Operator : Logic  Inputs=3  AllPortsSameDT=off  OutDataTypeStr=boolean
  Rate Transition : RateTransition  OutPortSampleTime=.001
  Rate Transition1 : RateTransition
  Switch : Switch  Criteria=u2 > Threshold  ZeroCross=off
  PCmd : Outport
  wires:
  Bang-bang controller/1(out_1) -> Gain/1
  Add/1 -> Bang-bang controller/1(in_1)
  Rate Transition1/1 -> PCmd/1
  <Kappa>/1 -> Rate Transition/1
  Pref/1 -> Switch/3, Compare To Constant1/1  "Pref"
  Constant/1 -> Add/2  "slip ref"
  Switch/1 -> Rate Transition1/1
  Rate Transition/1 -> Add/1, Compare To Constant/1
  Logical Operator/1 -> Debounce/1
  Compare To Constant/1 -> Logical Operator/2
  Compare To Constant1/1 -> Logical Operator/3
  Debounce/1 -> Switch/2
  xdot/1 -> Abs/1
  Abs/1 -> Compare To Constant2/1
  Compare To Constant2/1 -> Logical Operator/1
  Gain/1 -> Switch/1

== system MPC_control/Controllers/Brake Controller/Brake Pressure Control/Open Loop ==
  Pref : Inport
  PCmd : Outport
  wires:
  Pref/1 -> PCmd/1  "Reference Slip"

== system MPC_control/Controllers/Transmission Controller/TCM/Neutral Select ==
  AccCmd : Inport
  EngSpd : Inport  Port=2
  Constant : Constant  Value=1200
  Constant1 : Constant  Value=1e-6
  Logical Operator : Logic  AllPortsSameDT=off  OutDataTypeStr=boolean
  Relational Operator : RelationalOperator  Operator=<=  OutDataTypeStr=boolean  RndMeth=Simplest
  Relational Operator1 : RelationalOperator  Operator=<=  OutDataTypeStr=boolean  RndMeth=Simplest
  Saturation1 : Saturate  UpperLimit=10e3  LowerLimit=0
  rad/s to RPM : Gain  Gain=30/pi
  Neutral Select : Outport
  wires:
  Saturation1/1 -> Relational Operator/1
  Relational Operator1/1 -> Logical Operator/1
  AccCmd/1 -> Relational Operator1/1
  Constant1/1 -> Relational Operator1/2
  Logical Operator/1 -> Neutral Select/1
  Constant/1 -> Relational Operator/2
  Relational Operator/1 -> Logical Operator/2
  rad/s to RPM/1 -> Saturation1/1
  EngSpd/1 -> rad/s to RPM/1

== system MPC_control/Controllers/Transmission Controller/TCM/TCM Shift Controller/calc ==
  note: Determine if next gear will be
      | higher or lower than current gear
  gear : Inport
  pedal : Inport  Port=2
  speed : Inport  Port=3
  f : TriggerPort  TriggerType=function-call  VariantControl=Variant  StatesWhenEnabling=reset
      settings: CopyFcn=Stateflow.SLINSF.SimulinkMan.removeBlockPreDeleteFcn  PreDeleteFcn=Stateflow.SLINSF.SimulinkMan.unsafePredeleteFcn
  Add1 : Sum  Inputs=+-
  Add3 : Sum  Inputs=+-
  Add4 : Sum  Inputs=+-
  Calculate Upshift Threshold : Lookup_n-D  BreakpointsForDimension1=Pedal_Positions  BreakpointsForDimension2=1:7  Table=Upshift_Speeds  ExtrapMethod=Clip  UseLastTableValue=on  InternalRulePriority=Speed  RndMeth=Simplest  InputSameDT=on
  Calculate Downshift Threshold : Lookup_n-D  BreakpointsForDimension1=Pedal_Positions  BreakpointsForDimension2=2:8  Table=Downshift_Speeds  ExtrapMethod=Clip  UseLastTableValue=on  InternalRulePriority=Speed  RndMeth=Simplest  InputSameDT=on
  SpdThr : Outport
  wires:
  pedal/1 -> Calculate Downshift Threshold/1, Calculate Upshift Threshold/1
  gear/1 -> Calculate Downshift Threshold/2, Calculate Upshift Threshold/2
  Calculate Downshift Threshold/1 -> Add3/2
  Calculate Upshift Threshold/1 -> Add1/1
  speed/1 -> Add1/2, Add3/1
  Add1/1 -> Add4/1
  Add3/1 -> Add4/2
  Add4/1 -> SpdThr/1

== system MPC_control/Controllers/Transmission Controller/TCM/TCM Shift Controller/calc_down ==
  gear : Inport
  pedal : Inport  Port=2
  f : TriggerPort  TriggerType=function-call  VariantControl=Variant  StatesWhenEnabling=reset
      settings: CopyFcn=Stateflow.SLINSF.SimulinkMan.removeBlockPreDeleteFcn  PreDeleteFcn=Stateflow.SLINSF.SimulinkMan.unsafePredeleteFcn
  Calculate Downshift Threshold : Lookup_n-D  BreakpointsForDimension1=Pedal_Positions  BreakpointsForDimension2=2:8  Table=Downshift_Speeds  ExtrapMethod=Clip  UseLastTableValue=on  InternalRulePriority=Speed  RndMeth=Simplest  InputSameDT=on
  down_th : Outport
  wires:
  Calculate Downshift Threshold/1 -> down_th/1
  gear/1 -> Calculate Downshift Threshold/2
  pedal/1 -> Calculate Downshift Threshold/1

== system MPC_control/Controllers/Transmission Controller/TCM/TCM Shift Controller/calc_up ==
  gear : Inport
  pedal : Inport  Port=2
  f : TriggerPort  TriggerType=function-call  VariantControl=Variant  StatesWhenEnabling=reset
      settings: CopyFcn=Stateflow.SLINSF.SimulinkMan.removeBlockPreDeleteFcn  PreDeleteFcn=Stateflow.SLINSF.SimulinkMan.unsafePredeleteFcn
  Calculate Upshift Threshold : Lookup_n-D  BreakpointsForDimension1=Pedal_Positions  BreakpointsForDimension2=1:7  Table=Upshift_Speeds  ExtrapMethod=Clip  UseLastTableValue=on  InternalRulePriority=Speed  RndMeth=Simplest  InputSameDT=on
  up_th : Outport
  wires:
  Calculate Upshift Threshold/1 -> up_th/1
  pedal/1 -> Calculate Upshift Threshold/1
  gear/1 -> Calculate Upshift Threshold/2

== system MPC_control/Visualization/3D Engine/3D Engine/Part Rotation Concatenation ==
  Body Roll : Inport
  Body Ptich : Inport  Port=2
  Body Yaw : Inport  Port=3
  WheelFrontLeft Pitch : Inport  Port=4
  WheelFrontRight Pitch : Inport  Port=5
  WheelRearLeft Pitch : Inport  Port=6
  WheelRearRight Ptich : Inport  Port=7
  WheelFrontLeft Roll : Inport  Port=8
  WheelFrontRight Roll : Inport  Port=9
  WheelRearLeft Roll : Inport  Port=10
  WheelRearRight Roll : Inport  Port=11
  WheelFrontLeft Yaw : Inport  Port=12
  WheelFrontRight Yaw : Inport  Port=13
  WheelRearLeft Yaw : Inport  Port=14
  WheelRearRight Yaw : Inport  Port=15
  AllParts : Concatenate  NumInputs=5  Mode=Multidimensional array
  Body : Concatenate  NumInputs=3  Mode=Multidimensional array  ConcatenateDimension=2
  WheelFrontLeft : Concatenate  NumInputs=3  Mode=Multidimensional array  ConcatenateDimension=2
  WheelFrontRight : Concatenate  NumInputs=3  Mode=Multidimensional array  ConcatenateDimension=2
  WheelRearLeft : Concatenate  NumInputs=3  Mode=Multidimensional array  ConcatenateDimension=2
  WheelRearRight : Concatenate  NumInputs=3  Mode=Multidimensional array  ConcatenateDimension=2
  ConcatOut : Outport
  wires:
  Body Ptich/1 -> Body/1
  Body Yaw/1 -> Body/3
  WheelFrontLeft Pitch/1 -> WheelFrontLeft/1
  WheelFrontLeft Yaw/1 -> WheelFrontLeft/3
  WheelFrontLeft Roll/1 -> WheelFrontLeft/2
  Body Roll/1 -> Body/2
  WheelFrontLeft/1 -> AllParts/2
  WheelRearRight Ptich/1 -> WheelRearRight/1
  Body/1 -> AllParts/1
  WheelRearLeft/1 -> AllParts/4
  WheelFrontRight/1 -> AllParts/3
  WheelRearRight Yaw/1 -> WheelRearRight/3
  WheelFrontRight Roll/1 -> WheelFrontRight/2
  WheelFrontRight Pitch/1 -> WheelFrontRight/1
  WheelRearRight Roll/1 -> WheelRearRight/2
  WheelRearLeft Yaw/1 -> WheelRearLeft/3
  AllParts/1 -> ConcatOut/1
  WheelRearLeft Roll/1 -> WheelRearLeft/2
  WheelRearRight/1 -> AllParts/5
  WheelRearLeft Pitch/1 -> WheelRearLeft/1
  WheelFrontRight Yaw/1 -> WheelFrontRight/3

== system MPC_control/Visualization/3D Engine/3D Engine/Part Translation Concatenation ==
  BodyX : Inport
  BodyY : Inport  Port=2
  BodyZ : Inport  Port=3
  WheelFrontLeftX : Inport  Port=4
  WheelFrontRightX : Inport  Port=5
  WheelRearLeftX : Inport  Port=6
  WheelRearRightX : Inport  Port=7
  WheelFrontLeftY : Inport  Port=8
  WheelFrontRightY : Inport  Port=9
  WheelRearLeftY : Inport  Port=10
  WheelRearRightY : Inport  Port=11
  WheelFrontLeftZ : Inport  Port=12
  WheelFrontRightZ : Inport  Port=13
  WheelRearLeftZ : Inport  Port=14
  WheelRearRightZ : Inport  Port=15
  AllParts : Concatenate  NumInputs=5  Mode=Multidimensional array
  Body : Concatenate  NumInputs=3  Mode=Multidimensional array  ConcatenateDimension=2
  WheelFrontLeft : Concatenate  NumInputs=3  Mode=Multidimensional array  ConcatenateDimension=2
  WheelFrontRight : Concatenate  NumInputs=3  Mode=Multidimensional array  ConcatenateDimension=2
  WheelRearLeft : Concatenate  NumInputs=3  Mode=Multidimensional array  ConcatenateDimension=2
  WheelRearRight : Concatenate  NumInputs=3  Mode=Multidimensional array  ConcatenateDimension=2
  ConcatOut : Outport
  wires:
  BodyX/1 -> Body/1
  BodyZ/1 -> Body/3
  WheelFrontLeftX/1 -> WheelFrontLeft/1
  WheelFrontLeftZ/1 -> WheelFrontLeft/3
  WheelFrontLeftY/1 -> WheelFrontLeft/2
  BodyY/1 -> Body/2
  WheelFrontLeft/1 -> AllParts/2
  WheelRearRightX/1 -> WheelRearRight/1
  Body/1 -> AllParts/1
  WheelRearLeft/1 -> AllParts/4
  WheelFrontRight/1 -> AllParts/3
  WheelRearRightZ/1 -> WheelRearRight/3
  WheelFrontRightY/1 -> WheelFrontRight/2
  WheelFrontRightX/1 -> WheelFrontRight/1
  WheelRearRightY/1 -> WheelRearRight/2
  WheelRearLeftZ/1 -> WheelRearLeft/3
  AllParts/1 -> ConcatOut/1
  WheelRearLeftY/1 -> WheelRearLeft/2
  WheelRearRight/1 -> AllParts/5
  WheelRearLeftX/1 -> WheelRearLeft/1
  WheelFrontRightZ/1 -> WheelFrontRight/3

== system MPC_control/Visualization/3D Engine/3D Engine/Scale ==
  Constant{1..12,17,32..33} (15 alike) : Constant  OutDataTypeStr=single
  PartConcatenation : Subsystem
  ScaleOut : Outport
  wires:
  Constant10/1 -> PartConcatenation/15(WheelRearRightZ)
  Constant9/1 -> PartConcatenation/14(WheelRearRightY)
  Constant11/1 -> PartConcatenation/13(WheelRearRightX)
  Constant7/1 -> PartConcatenation/12(WheelRearLeftZ)
  Constant6/1 -> PartConcatenation/11(WheelRearLeftY)
  Constant8/1 -> PartConcatenation/10(WheelRearLeftX)
  Constant4/1 -> PartConcatenation/9(WheelFrontRightZ)
  Constant3/1 -> PartConcatenation/8(WheelFrontRightY)
  Constant5/1 -> PartConcatenation/7(WheelFrontRightX)
  Constant2/1 -> PartConcatenation/6(WheelFrontLeftZ)
  Constant1/1 -> PartConcatenation/5(WheelFrontLeftY)
  Constant33/1 -> PartConcatenation/4(WheelFrontLeftX)
  Constant32/1 -> PartConcatenation/3(BodyZ)
  Constant17/1 -> PartConcatenation/2(BodyY)
  Constant12/1 -> PartConcatenation/1(BodyX)
  PartConcatenation/1(ConcatOut) -> ScaleOut/1

== system MPC_control/observer_of_plant/Subsystem_1/simulator_1/MPC_of_simulator_1 ==
  Velocity_updated : Inport  SampleTime=Ts  LockScale=on
  Heading_updated : Inport  Port=2  SampleTime=Ts  LockScale=on
  Xhat : Inport  Port=3
  U(k-1) : Inport  Port=4  SampleTime=Ts  LockScale=on
  select_MPC : Inport  Port=5  SampleTime=Ts  LockScale=on
  select_overlap : Inport  Port=6  SampleTime=Ts  LockScale=on
  Clock : Clock
  Constant1 : Constant  Value=M  VectorParams1D=off  SampleTime=-1
  Constant2 : Constant  Value=Np  SampleTime=-1
  Constant3 : Constant  Value=JE_1  VectorParams1D=off  SampleTime=-1
  Constant4 : Constant  Value=Qc_1  VectorParams1D=off  SampleTime=-1
  Constant5 : Constant  Value=phi_1  VectorParams1D=off  SampleTime=-1
  F_Middle : Gain  Gain=F_1  Multiplication=Matrix(K*u) (u vector)
  From Workspace6 : FromWorkspace  VariableName=Rs  SampleTime=Ts
  HQP : MATLAB Function  TreatAsAtomicUnit=on  SystemSampleTime=Ts
  Resettable Delay2 : Delay  DelayLength=1  InitialConditionSource=Input port  ExternalReset=Rising  SampleTime=Ts
      settings: InputPortMap=u0,r5,p4
  r(k+1) : Outport
  U : Outport  Port=2
  wires:
  HQP/2(U) -> Resettable Delay2/1, U/1
  Xhat/1 -> F_Middle/1
  Constant4/1 -> HQP/4(Qc)
  Constant5/1 -> HQP/2(phi)
  Constant3/1 -> HQP/1(JE)
  Constant2/1 -> HQP/6(Np)
  Constant1/1 -> HQP/5(M)
  Clock/1 -> HQP/10(Tsim)
  F_Middle/1 -> HQP/3(Fxh)
  From Workspace6/1 -> HQP/9(Rs)
  Heading_updated/1 -> HQP/7(Heading_updated)
  Velocity_updated/1 -> HQP/8(Velocity_updated)
  HQP/1(r) -> r(k+1)/1
  select_MPC/1 -> HQP/11(select_MPC)
  Resettable Delay2/1 -> HQP/12(U_delay)
  select_overlap/1 -> Resettable Delay2/2
  U(k-1)/1 -> Resettable Delay2/3

== system MPC_control/observer_of_plant/Subsystem_1/simulator_1/VH2P ==
  Velocities : Inport
  HeadingAngles : Inport  Port=2
  Initial position : Inport  Port=3
  Iintial Velocities : Inport  Port=4
  Iintial HeadingAngles : Inport  Port=5
  select_overlap : Inport  Port=6
  From Workspace1 : FromWorkspace  VariableName=Tsim  SampleTime=Ts
  Resettable Delay1 : Delay  DelayLength=1  InitialConditionSource=Input port  ExternalReset=Rising  SampleTime=Ts
      settings: InputPortMap=u0,r5,p4
  Resettable Delay2 : Delay  DelayLength=1  InitialConditionSource=Input port  ExternalReset=Rising  SampleTime=Ts
      settings: InputPortMap=u0,r5,p4
  Resettable Delay3 : Delay  DelayLength=1  InitialConditionSource=Input port  ExternalReset=Rising  SampleTime=Ts
      settings: InputPortMap=u0,r5,p4
  Unit Delay2 : UnitDelay  SampleTime=Ts
  YV2P : MATLAB Function  TreatAsAtomicUnit=on  SystemSampleTime=Ts
  Position : Outport
  wires:
  YV2P/1(Position) -> Resettable Delay3/1, Position/1
  Velocities/1 -> Resettable Delay1/1, YV2P/1(Velocity)
  Resettable Delay1/1 -> YV2P/2(LastVelocity)
  HeadingAngles/1 -> Resettable Delay2/1, YV2P/3(Heading)
  Resettable Delay2/1 -> YV2P/4(LastHeading)
  Resettable Delay3/1 -> YV2P/7(Lastpostion)
  Initial position/1 -> Resettable Delay3/3
  Iintial Velocities/1 -> Resettable Delay1/3
  Iintial HeadingAngles/1 -> Resettable Delay2/3
  select_overlap/1 -> Resettable Delay3/2, Resettable Delay2/2, Resettable Delay1/2
  From Workspace1/1 -> YV2P/5(Tsim), Unit Delay2/1
  Unit Delay2/1 -> YV2P/6(LastTsim)

== system MPC_control/observer_of_plant/Subsystem_1/simulator_1/YV_update ==
  XY_sim : Inport
  Velocity_sim : Inport  Port=2
  Heading_sim : Inport  Port=3
  Constant : Constant  Value=Ts  SampleTime=Ts
  Discrete-Time Integrator : DiscreteIntegrator  Commented=on  SampleTime=Ts  ICPrevOutput=DiscIntNeverNeededParam  ICPrevScaledInput=DiscIntNeverNeededParam
  From Workspace1 : FromWorkspace  VariableName=Tsim  SampleTime=Ts
  From Workspace3 : FromWorkspace  VariableName=XYplot_ref  SampleTime=Ts
  Gain : Gain  Commented=on  Gain=[eye(2), zeros(2,10)]  Multiplication=Matrix(K*u) (u vector)
  Mux : Mux  Commented=on  Inputs=2
  Pure Pursuit : robotalgslib/Pure Pursuit  Commented=on  DesiredLinearVelocity=0.1  MaxAngularVelocity=1.0  LookaheadDistance=2.5  TargetDirPort=off  SimulateUsing=Code generation
      settings: SourceProductName=Robotics System Toolbox  SourceProductBaseCode=RO
  Transpose : Math  Commented=on  Operator=transpose  SaturateOnIntegerOverflow=on
  YV_update : MATLAB Function  TreatAsAtomicUnit=on  SystemSampleTime=Ts
  Velocity_updated : Outport
  Heading_updated : Outport  Port=2
  wires:
  From Workspace1/1 -> YV_update/6(Tsim)
  Velocity_sim/1 -> YV_update/3(Velocity_sim)
  Constant/1 -> YV_update/5(Ts)
  From Workspace3/1 -> Gain/1, YV_update/1(XYplot_ref)
  Pure Pursuit/2 -> Discrete-Time Integrator/1
  Heading_sim/1 -> Mux/2, YV_update/4(Heading_sim)
  Mux/1 -> Pure Pursuit/1
  YV_update/1(Velocity_updated) -> Velocity_updated/1
  XY_sim/1 -> Mux/1, YV_update/2(XYplot_sim)
  Gain/1 -> Transpose/1
  Transpose/1 -> Pure Pursuit/2
  YV_update/2(Heading_updated) -> Heading_updated/1

== system MPC_control/observer_of_plant/Subsystem_2/simulator_2/MPC_of_simulator_2 ==
  Velocity_updated : Inport  SampleTime=Ts  LockScale=on
  Heading_updated : Inport  Port=2  SampleTime=Ts  LockScale=on
  Xhat : Inport  Port=3
  U(k-1) : Inport  Port=4  SampleTime=Ts  LockScale=on
  select_MPC : Inport  Port=5  SampleTime=Ts  LockScale=on
  select_overlap : Inport  Port=6  SampleTime=Ts  LockScale=on
  Clock : Clock
  Constant1 : Constant  Value=M  VectorParams1D=off  SampleTime=-1
  Constant2 : Constant  Value=Np  SampleTime=-1
  Constant3 : Constant  Value=JE_2  VectorParams1D=off  SampleTime=-1
  Constant4 : Constant  Value=Qc_2  VectorParams1D=off  SampleTime=-1
  Constant5 : Constant  Value=phi_2  VectorParams1D=off  SampleTime=-1
  F_Middle : Gain  Gain=F_2  Multiplication=Matrix(K*u) (u vector)
  From Workspace6 : FromWorkspace  VariableName=Rs  SampleTime=Ts
  HQP : MATLAB Function  TreatAsAtomicUnit=on  SystemSampleTime=Ts
  Resettable Delay2 : Delay  DelayLength=1  InitialConditionSource=Input port  ExternalReset=Rising  SampleTime=Ts
      settings: InputPortMap=u0,r5,p4
  r(k+1) : Outport
  U : Outport  Port=2
  wires:
  HQP/2(U) -> Resettable Delay2/1, U/1
  Xhat/1 -> F_Middle/1
  Constant4/1 -> HQP/4(Qc)
  Constant5/1 -> HQP/2(phi)
  Constant3/1 -> HQP/1(JE)
  Constant2/1 -> HQP/6(Np)
  Constant1/1 -> HQP/5(M)
  Clock/1 -> HQP/10(Tsim)
  F_Middle/1 -> HQP/3(Fxh)
  From Workspace6/1 -> HQP/9(Rs)
  Heading_updated/1 -> HQP/7(Heading_updated)
  Velocity_updated/1 -> HQP/8(Velocity_updated)
  HQP/1(r) -> r(k+1)/1
  select_MPC/1 -> HQP/11(select_MPC)
  Resettable Delay2/1 -> HQP/12(U_delay)
  select_overlap/1 -> Resettable Delay2/2
  U(k-1)/1 -> Resettable Delay2/3

== system MPC_control/observer_of_plant/Subsystem_2/simulator_2/VH2P ==
  Velocities : Inport
  HeadingAngles : Inport  Port=2
  Initial position : Inport  Port=3
  Iintial Velocities : Inport  Port=4
  Iintial HeadingAngles : Inport  Port=5
  select_overlap : Inport  Port=6
  From Workspace1 : FromWorkspace  VariableName=Tsim  SampleTime=Ts
  Resettable Delay1 : Delay  DelayLength=1  InitialConditionSource=Input port  ExternalReset=Rising  SampleTime=Ts
      settings: InputPortMap=u0,r5,p4
  Resettable Delay2 : Delay  DelayLength=1  InitialConditionSource=Input port  ExternalReset=Rising  SampleTime=Ts
      settings: InputPortMap=u0,r5,p4
  Resettable Delay3 : Delay  DelayLength=1  InitialConditionSource=Input port  ExternalReset=Rising  SampleTime=Ts
      settings: InputPortMap=u0,r5,p4
  Unit Delay2 : UnitDelay  SampleTime=Ts
  YV2P : MATLAB Function  TreatAsAtomicUnit=on  SystemSampleTime=Ts
  Position : Outport
  wires:
  YV2P/1(Position) -> Resettable Delay3/1, Position/1
  Velocities/1 -> Resettable Delay1/1, YV2P/1(Velocity)
  Resettable Delay1/1 -> YV2P/2(LastVelocity)
  HeadingAngles/1 -> Resettable Delay2/1, YV2P/3(Heading)
  Resettable Delay2/1 -> YV2P/4(LastHeading)
  Resettable Delay3/1 -> YV2P/7(Lastpostion)
  Initial position/1 -> Resettable Delay3/3
  Iintial Velocities/1 -> Resettable Delay1/3
  Iintial HeadingAngles/1 -> Resettable Delay2/3
  select_overlap/1 -> Resettable Delay3/2, Resettable Delay2/2, Resettable Delay1/2
  From Workspace1/1 -> YV2P/5(Tsim), Unit Delay2/1
  Unit Delay2/1 -> YV2P/6(LastTsim)

== system MPC_control/observer_of_plant/Subsystem_2/simulator_2/YV_update ==
  XY_sim : Inport
  Velocity_sim : Inport  Port=2
  Heading_sim : Inport  Port=3
  Constant : Constant  Value=Ts  SampleTime=Ts
  Discrete-Time Integrator : DiscreteIntegrator  Commented=on  SampleTime=Ts  ICPrevOutput=DiscIntNeverNeededParam  ICPrevScaledInput=DiscIntNeverNeededParam
  From Workspace1 : FromWorkspace  VariableName=Tsim  SampleTime=Ts
  From Workspace3 : FromWorkspace  VariableName=XYplot_ref  SampleTime=Ts
  Gain : Gain  Commented=on  Gain=[eye(2), zeros(2,10)]  Multiplication=Matrix(K*u) (u vector)
  Mux : Mux  Commented=on  Inputs=2
  Pure Pursuit : robotalgslib/Pure Pursuit  Commented=on  DesiredLinearVelocity=0.1  MaxAngularVelocity=1.0  LookaheadDistance=2.5  TargetDirPort=off  SimulateUsing=Code generation
      settings: SourceProductName=Robotics System Toolbox  SourceProductBaseCode=RO
  Transpose : Math  Commented=on  Operator=transpose  SaturateOnIntegerOverflow=on
  YV_update : MATLAB Function  TreatAsAtomicUnit=on  SystemSampleTime=Ts
  Velocity_updated : Outport
  Heading_updated : Outport  Port=2
  wires:
  YV_update/1(Velocity_updated) -> Velocity_updated/1
  From Workspace1/1 -> YV_update/6(Tsim)
  Velocity_sim/1 -> YV_update/3(Velocity_sim)
  Constant/1 -> YV_update/5(Ts)
  XY_sim/1 -> Mux/1, YV_update/2(XYplot_sim)
  From Workspace3/1 -> Gain/1, YV_update/1(XYplot_ref)
  Pure Pursuit/2 -> Discrete-Time Integrator/1
  Heading_sim/1 -> Mux/2, YV_update/4(Heading_sim)
  Mux/1 -> Pure Pursuit/1
  Gain/1 -> Transpose/1
  Transpose/1 -> Pure Pursuit/2
  YV_update/2(Heading_updated) -> Heading_updated/1

== system MPC_control/observer_of_plant/Subsystem_3/simulator_3/MPC_of_simulator_3 ==
  Velocity_updated : Inport  SampleTime=Ts  LockScale=on
  Heading_updated : Inport  Port=2  SampleTime=Ts  LockScale=on
  Xhat : Inport  Port=3
  U(k-1) : Inport  Port=4  SampleTime=Ts  LockScale=on
  select_MPC : Inport  Port=5  SampleTime=Ts  LockScale=on
  select_overlap : Inport  Port=6  SampleTime=Ts  LockScale=on
  Clock : Clock
  Constant1 : Constant  Value=M  VectorParams1D=off  SampleTime=-1
  Constant2 : Constant  Value=Np  SampleTime=-1
  Constant3 : Constant  Value=JE_3  VectorParams1D=off  SampleTime=-1
  Constant4 : Constant  Value=Qc_3  VectorParams1D=off  SampleTime=-1
  Constant5 : Constant  Value=phi_3  VectorParams1D=off  SampleTime=-1
  F_Middle : Gain  Gain=F_3  Multiplication=Matrix(K*u) (u vector)
  From Workspace6 : FromWorkspace  VariableName=Rs  SampleTime=Ts
  HQP : MATLAB Function  TreatAsAtomicUnit=on  SystemSampleTime=Ts
  Resettable Delay2 : Delay  DelayLength=1  InitialConditionSource=Input port  ExternalReset=Rising  SampleTime=Ts
      settings: InputPortMap=u0,r5,p4
  r(k+1) : Outport
  U : Outport  Port=2
  wires:
  HQP/2(U) -> Resettable Delay2/1, U/1
  Xhat/1 -> F_Middle/1
  Constant4/1 -> HQP/4(Qc)
  Constant5/1 -> HQP/2(phi)
  Constant3/1 -> HQP/1(JE)
  Constant2/1 -> HQP/6(Np)
  Constant1/1 -> HQP/5(M)
  Clock/1 -> HQP/10(Tsim)
  F_Middle/1 -> HQP/3(Fxh)
  From Workspace6/1 -> HQP/9(Rs)
  Heading_updated/1 -> HQP/7(Heading_updated)
  Velocity_updated/1 -> HQP/8(Velocity_updated)
  HQP/1(r) -> r(k+1)/1
  select_MPC/1 -> HQP/11(select_MPC)
  Resettable Delay2/1 -> HQP/12(U_delay)
  select_overlap/1 -> Resettable Delay2/2
  U(k-1)/1 -> Resettable Delay2/3
